simulink model "usato"  (R2016a)
settings: Solver=ode3  StartTime=0.0  StopTime=200  FixedStep=0.1  RelTol=1e-5
values from neighbouring files (symbols this model uses):
  c = 0.1    [Script.m]
  Kd = 0.9    [Script.m]
  Ki = 0.036    [Script.m]
  Kp = 0.37    [Script.m]
  N = 5    [Script.m]
libraries: simulink x2
(part 1 of 2)
settings Model: Creator=The MathWorks, Inc.  LastModifiedBy=User
settings SolverCC: MaxConsecutiveZCs=100000  ZeroCrossAlgorithm=Adaptive
settings DataIOCC: MaxDataPoints=100000  SaveFormat=Array
settings OptimizationCC: ExpressionDepthLimit=2147483647
settings DebuggingCC: UnderspecifiedInitializationDetection=Classic  MergeDetectMultiDrivingBlocksExec=none  FcnCallInpInsideContextMsg=UseLocalSettings  StateNameClashWarn=warning
settings HardwareCC: ProdBitPerPointer=32  ProdLargestAtomicFloat=None  ProdIntDivRoundTo=Undefined  ProdEndianess=Unspecified  ProdWordSize=32  ProdHWDeviceType=32-bit Generic
settings ModelReferenceCC: PropagateSignalLabelsOutOfModel=off
settings GRTTargetCC: CombineOutputUpdateFcns=off  GRTInterface=on
settings ConfigComp: CovModelRefEnable=Off

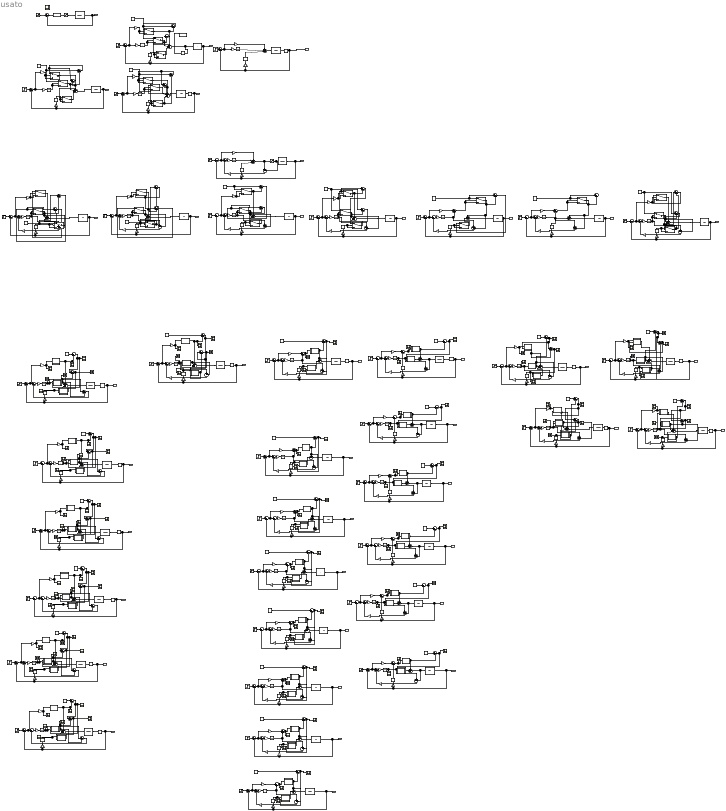
== system usato ==
  note: DESATURAZIONE CLASSICA
  note: TASK P, poi I,poi D
  note: TASK I,poi P,poi D
  note: PI
  note: Anti-Windup PID Control Demonstration
  note: TASK D, poi P,poi I
  note: TASK P, poi D, poi I
  note: TASK I,poi D,poi P
  note: TASK D, poi I,poi P
  note: PD
  note: TASK P, poi I, poi D k=1
  note: PI k=1
  note: PD K=1
  note: TASK I,poi P,poi D
  note: TASK I,poi D,poi P
  note: TASK D, poi P,poi I
  note: TASK D, poi I,poi D
  note: PI k=0.1
  note: PI k=2.8
  note: PI k=2
  note: PI k=3
  note: PI k=0.5
  note: PI k=0.2
  note: PI k=0.75
  note: TASK P, poi I, poi D k=0.1
  note: TASK P, poi I, poi D k=0.2
  note: TASK P, poi I, poi D k=0.5
  note: TASK P, poi I, poi D k=2
  note: TASK P, poi I, poi D k=1,5
  note: PD K=0.1
  note: PD K=0.01
  note: PD K=3
  note: PD K=0.3
  note: PD K=0.03
  C1(t){,1..5} (6 alike) : Constant  Value=c
  Constant{,5..6,10,13..15} (7 alike) : Constant  Value=1.05
  Constant1 : Constant  Value=1.5
  Constant{2,7..9,11..12,16..22} (13 alike) : Constant  Value=c
  Constant3 : Constant  Value=0.1
  Constant4 : Constant  Value=10
  DERIVATIVE{1..37} (37 alike) : Derivative
  Dead Time{,1..14} (15 alike) : TransportDelay  BufferSize=2048
  First Order Process{,2..4,10..12,14..15,19..20} (11 alike) : TransferFcn  Numerator=1  Denominator=[1 1 0]
  First Order Process{1,6,9,16,18} (5 alike) : TransferFcn  Numerator=1  Denominator=[1 0 0]
  First Order Process{5,7,13,17} (4 alike) : TransferFcn  Numerator=1  Denominator=[1 0]
  First Order Process21 : TransferFcn  Numerator=0.1  Denominator=[1 0]
  First Order Process22 : TransferFcn  Numerator=2.8  Denominator=[1 0]
  First Order Process23 : TransferFcn  Numerator=2  Denominator=[1 0]
  First Order Process24 : TransferFcn  Numerator=3  Denominator=[1 0]
  First Order Process25 : TransferFcn  Numerator=0.5  Denominator=[1 0]
  First Order Process26 : TransferFcn  Numerator=0.2  Denominator=[1 0]
  First Order Process27 : TransferFcn  Numerator=0.75  Denominator=[1 0]
  First Order Process28 : TransferFcn  Numerator=0.1  Denominator=[1 1 0]
  First Order Process29 : TransferFcn  Numerator=0.2  Denominator=[1 1 0]
  First Order Process30 : TransferFcn  Numerator=0.5  Denominator=[1 1 0]
  First Order Process31 : TransferFcn  Numerator=2  Denominator=[1 1 0]
  First Order Process32 : TransferFcn  Numerator=1.5  Denominator=[1 1 0]
  First Order Process33 : TransferFcn  Numerator=0.1  Denominator=[1 0 0]
  First Order Process34 : TransferFcn  Numerator=0.01  Denominator=[1 0 0]
  First Order Process35 : TransferFcn  Numerator=3  Denominator=[1 0 0]
  First Order Process36 : TransferFcn  Numerator=100  Denominator=[1 0 0]
  First Order Process37 : TransferFcn  Numerator=0.03  Denominator=[1 0 0]
  First Order Process8 : TransferFcn  Numerator=1  Denominator=[1 1]
  INTEGRATOR{1..25} (25 alike) : Integrator
  Integrator{,1..5} (6 alike) : Integrator
  Kd{1,8,13,17} (4 alike) : Gain  Gain=0
  Kd{4..5,10..12,14..15,19..31} (20 alike) : Gain  Gain=Kd
  Kd{6..7,9,16,18} (5 alike) : Gain  Gain=10
  Kd2 : Gain  Gain=0.9
  Kd3 : Gain  Gain=0.9
  Ki{1,6..9,13,16..18} (9 alike) : Gain  Gain=10
  Ki{4..5,10..12,14..15,19..31} (20 alike) : Gain  Gain=Ki
  Ki2 : Gain  Gain=0.036
  Ki3 : Gain  Gain=0.036
  Kp{1,6..9,13,16..18} (9 alike) : Gain  Gain=10
  Kp{4..5,10..12,14..15,19..31} (20 alike) : Gain  Gain=Kp
  Kp2 : Gain  Gain=0.37
  Kp3 : Gain  Gain=0.37
  MATLAB Function : MATLAB Function  TreatAsAtomicUnit=on
  MATLAB Function1 : MATLAB Function  TreatAsAtomicUnit=on
  MATLAB Function10 : MATLAB Function  TreatAsAtomicUnit=on
  MATLAB Function11 : MATLAB Function  TreatAsAtomicUnit=on
  MATLAB Function12 : MATLAB Function  TreatAsAtomicUnit=on
  MATLAB Function13 : MATLAB Function  TreatAsAtomicUnit=on
  MATLAB Function14 : MATLAB Function  TreatAsAtomicUnit=on
  MATLAB Function15 : MATLAB Function  TreatAsAtomicUnit=on
  MATLAB Function16 : MATLAB Function  TreatAsAtomicUnit=on
  MATLAB Function17 : MATLAB Function  TreatAsAtomicUnit=on
  MATLAB Function18 : MATLAB Function  TreatAsAtomicUnit=on
  MATLAB Function19 : MATLAB Function  TreatAsAtomicUnit=on
  MATLAB Function2 : MATLAB Function  TreatAsAtomicUnit=on
  MATLAB Function20 : MATLAB Function  TreatAsAtomicUnit=on
  MATLAB Function3 : MATLAB Function  TreatAsAtomicUnit=on
  MATLAB Function4 : MATLAB Function  TreatAsAtomicUnit=on
  MATLAB Function5 : MATLAB Function  TreatAsAtomicUnit=on
  MATLAB Function6 : MATLAB Function  TreatAsAtomicUnit=on
  MATLAB Function7 : MATLAB Function  TreatAsAtomicUnit=on
  MATLAB Function8 : MATLAB Function  TreatAsAtomicUnit=on
  MATLAB Function9 : MATLAB Function  TreatAsAtomicUnit=on
  Memory : Memory
  MinMax Running Resettable : simulink/Math Operations/MinMax Running Resettable  Function=max  vinit=0.0
  PID Controller : simulink/Continuous/PID Controller  Controller=PID  TimeDomain=Continuous-time  SampleTime=-1  IntegratorMethod=Forward Euler  FilterMethod=Forward Euler  Form=Parallel  UseFilter=on  ControllerParametersSource=internal  P=Kp  I=Ki  D=Kd  N=N  InitialConditionSource=internal  InitialConditionForIntegrator=0  InitialConditionForFilter=0  ExternalReset=none  LimitOutput=off  UpperSaturationLimit=10  LowerSaturationLimit=-10  LinearizeAsGain=off  AntiWindupMode=none  Kb=1  TrackingMode=off  Kt=1  PParamMin=[]  PParamMax=[]  IParamMin=[]  IParamMax=[]  DParamMin=[]  DParamMax=[]  NParamMin=[]  NParamMax=[]  KbParamMin=[]  KbParamMax=[]  KtParamMin=[]  KtParamMax=[]  POutMin=[]  POutMax=[]  IOutMin=[]  IOutMax=[]  DOutMin=[]  DOutMax=[]  NOutMin=[]  NOutMax=[]  KbOutMin=[]  KbOutMax=[]  KtOutMin=[]  KtOutMax=[]  IntegratorOutMin=[]  IntegratorOutMax=[]  FilterOutMin=[]  FilterOutMax=[]  SumOutMin=[]  SumOutMax=[]  SumI1OutMin=[]  SumI1OutMax=[]  SumI2OutMin=[]  SumI2OutMax=[]  SumI3OutMin=[]  SumI3OutMax=[]  SumDOutMin=[]  SumDOutMax=[]  SaturationOutMin=[]  SaturationOutMax=[]  IntegratorContinuousStateAttributes=''  IntegratorStateMustResolveToSignalObject=off  IntegratorRTWStateStorageClass=Auto  FilterContinuousStateAttributes=''  FilterStateMustResolveToSignalObject=off  FilterRTWStateStorageClass=Auto  DifferentiatorICPrevScaledInput=0  DifferentiatorOutMin=[]  DifferentiatorOutMax=[]
  Saturation : Saturate  UpperLimit=c  LowerLimit=-c
  Saturation1 : Saturate  UpperLimit=c  LowerLimit=-c
  Scope{,1..69} (70 alike) : Scope
  Step{,1..31} (32 alike) : Step  SampleTime=0
  Sum{,1..4,6..10,13..15,17,19..21,23..27,29..31,33..37,39,41,43..45,47..51,53..57,59..61,63..67,69..73,75..79,81..85,87..91,93..99,101..105,107..108,110,112..114,116,118..120,122,124..126,128,130..132,134,136..138,140,142..144,146,148..153,155..159,161..165,167..171,173..177,179..183,185..189,191..195,197..201,203..207,209..210} (165 alike) : Sum  Inputs=|+-
  Sum{5,12,16,18,22,28,32,52,58,62,68,74,80,86,100,106,154,160,166,172,178} (21 alike) : Sum  Inputs=++-|
  Sum{11,38,109,115,121,127,133,139,145} (9 alike) : Sum  Inputs=+-|
  Sum{40,42,111,117,123,129,135,141,147} (9 alike) : Sum  Inputs=|++
  Sum{46,92,184,190,196,202,208} (7 alike) : Sum  Inputs=++|
  Switch{,1..2,9..11,15..17,19..20,28..30,36..41,43} (21 alike) : Switch  Threshold=1.05
  Switch12 : Switch  Threshold=10
  Switch13 : Switch  Threshold=10
  Switch14 : Switch  Threshold=10
  Switch3 : Switch  Threshold=1.5
  Switch4 : Switch  Threshold=1.5
  Switch5 : Switch  Threshold=1.5
  c1(t){,1..5} (6 alike) : Constant  Value=c
  integratore{,1..5} (6 alike) : Integrator
  ka{,1..26} (27 alike) : Gain
  kd{,1..5} (6 alike) : Gain  Gain=Kd
  ki{,1..5} (6 alike) : Gain  Gain=Ki
  kp{,1..5} (6 alike) : Gain  Gain=Kp
  scope{1..42} (42 alike) : Scope
  sigma1 dpi : MATLAB Function  TreatAsAtomicUnit=on
  sigma1 dpi1 : MATLAB Function  TreatAsAtomicUnit=on
  sigma1 idp : MATLAB Function  TreatAsAtomicUnit=on
  sigma1 ipd : MATLAB Function  TreatAsAtomicUnit=on
  sigma1 pd : MATLAB Function  TreatAsAtomicUnit=on
  sigma1 pd1 : MATLAB Function  TreatAsAtomicUnit=on
  sigma1 pd2 : MATLAB Function  TreatAsAtomicUnit=on
  sigma1 pd3 : MATLAB Function  TreatAsAtomicUnit=on
  sigma1 pd4 : MATLAB Function  TreatAsAtomicUnit=on
  sigma1 pd5 : MATLAB Function  TreatAsAtomicUnit=on
  sigma1 pi : MATLAB Function  TreatAsAtomicUnit=on
  sigma1 pi1 : MATLAB Function  TreatAsAtomicUnit=on
  sigma1 pi2 : MATLAB Function  TreatAsAtomicUnit=on
  sigma1 pi3 : MATLAB Function  TreatAsAtomicUnit=on
  sigma1 pi4 : MATLAB Function  TreatAsAtomicUnit=on
  sigma1 pi5 : MATLAB Function  TreatAsAtomicUnit=on
  sigma1 pi6 : MATLAB Function  TreatAsAtomicUnit=on
  sigma1 pi7 : MATLAB Function  TreatAsAtomicUnit=on
  sigma2  idp : MATLAB Function  TreatAsAtomicUnit=on
  sigma2 dpi : MATLAB Function  TreatAsAtomicUnit=on
  sigma2 idp : MATLAB Function  TreatAsAtomicUnit=on
  sigma2 ipd : MATLAB Function  TreatAsAtomicUnit=on
  sigma2 pd : MATLAB Function  TreatAsAtomicUnit=on
  sigma2 pd1 : MATLAB Function  TreatAsAtomicUnit=on
  sigma2 pd2 : MATLAB Function  TreatAsAtomicUnit=on
  sigma2 pd3 : MATLAB Function  TreatAsAtomicUnit=on
  sigma2 pd4 : MATLAB Function  TreatAsAtomicUnit=on
  sigma2 pd5 : MATLAB Function  TreatAsAtomicUnit=on
  sigma2 pi : MATLAB Function  TreatAsAtomicUnit=on
  sigma2 pi1 : MATLAB Function  TreatAsAtomicUnit=on
  sigma2 pi2 : MATLAB Function  TreatAsAtomicUnit=on
  sigma2 pi3 : MATLAB Function  TreatAsAtomicUnit=on
  sigma2 pi4 : MATLAB Function  TreatAsAtomicUnit=on
  sigma2 pi5 : MATLAB Function  TreatAsAtomicUnit=on
  sigma2 pi6 : MATLAB Function  TreatAsAtomicUnit=on
  sigma2 pi7 : MATLAB Function  TreatAsAtomicUnit=on
  sigma3  idp : MATLAB Function  TreatAsAtomicUnit=on
  sigma3  idp1 : MATLAB Function  TreatAsAtomicUnit=on
  sigma3 dpi : MATLAB Function  TreatAsAtomicUnit=on
  sigma3 ipd : MATLAB Function  TreatAsAtomicUnit=on
  step{,1..5} (6 alike) : Step  SampleTime=0
  yout : Outport
  yout5 : Outport  Port=2
  yout2 : Outport  Port=3
  yout6 : Outport  Port=4
  yout1 : Outport  Port=5
  yout4 : Outport  Port=6
  yout7 : Outport  Port=7
  yout8 : Outport  Port=8
  yout9 : Outport  Port=9
  yout13 : Outport  Port=10
  yout14 : Outport  Port=11
  yout16 : Outport  Port=12
  yout17 : Outport  Port=13
  yout18 : Outport  Port=14
  yout15 : Outport  Port=15
  yout3 : Outport  Port=16
  yout10 : Outport  Port=17
  yout11 : Outport  Port=18
  yout20 : Outport  Port=19
  yout12 : Outport  Port=20
  yout19 : Outport  Port=21
  yout21 : Outport  Port=22
  yout22 : Outport  Port=23
  yout23 : Outport  Port=24
  yout24 : Outport  Port=25
  yout25 : Outport  Port=26
  yout26 : Outport  Port=27
  yout27 : Outport  Port=28
  yout28 : Outport  Port=29
  yout29 : Outport  Port=30
  yout30 : Outport  Port=31
  yout31 : Outport  Port=32
  yout32 : Outport  Port=33
  yout33 : Outport  Port=34
  yout34 : Outport  Port=35
  yout35 : Outport  Port=36
  yout36 : Outport  Port=37
  yout37 : Outport  Port=38
  wires:
  Step/1 -> Sum/1  "r(t)"
  Sum/1 -> PID Controller/1  "e(t)"
  First Order Process/1 -> yout/1, Sum/2  "y(t) con saturazione"
  Step5/1 -> Sum10/1  "r(t)"
  Sum10/1 -> Ki1/1, Kp1/1  "e(t)"
  First Order Process5/1 -> yout5/1, Kd1/1, Sum10/2  "yintegrat(t)"
  Ki1/1 -> INTEGRATOR1/1
  Kd1/1 -> DERIVATIVE1/1
  Kp1/1 -> Switch/3, Switch/2
  Switch/1 -> Sum1/2, Sum12/1
  Switch2/1 -> Sum12/3
  DERIVATIVE1/1 -> Switch2/2, Switch2/3
  INTEGRATOR1/1 -> Switch1/3, Switch1/2  "u(t)"
  Switch1/1 -> Sum2/2, Sum12/2
  Sum2/1 -> Switch2/1
  Step2/1 -> Sum14/1  "r(t)"
  Sum14/1 -> Ki3/1, Kp3/1  "e(t)"
  Ki3/1 -> INTEGRATOR3/1
  Kd3/1 -> DERIVATIVE3/1
  INTEGRATOR3/1 -> Sum16/2  "u(t)"
  Kp3/1 -> Sum16/1
  DERIVATIVE3/1 -> Sum16/3
  PID Controller/1 -> Saturation/1  "u(t)"
  Saturation/1 -> First Order Process/1
  Sum12/1 -> Memory/1, First Order Process5/1  "u(t)"
  Step6/1 -> Sum26/1  "r(t)"
  Sum26/1 -> Ki6/1, Kp6/1  "e(t)"
  First Order Process6/1 -> yout6/1, Kd6/1, Sum26/2  "yint(t)"
  Ki6/1 -> INTEGRATOR6/1
  Kd6/1 -> DERIVATIVE6/1
  Constant4/1 -> Switch13/1, Sum25/1
  Kp6/1 -> Switch12/3, Switch12/2
  Switch14/1 -> Sum28/3
  DERIVATIVE6/1 -> Switch14/2, Switch14/3
  INTEGRATOR6/1 -> Switch13/3, Switch13/2  "u(t)"
  Sum30/1 -> Switch14/1
  Sum25/1 -> Sum30/1, Switch12/1
  Switch13/1 -> Sum25/2, Sum28/2
  Switch12/1 -> Sum30/2, Sum28/1
  Sum28/1 -> First Order Process6/1  "u(t)"
  Step1/1 -> Sum4/1  "r(t)"
  Sum4/1 -> Ki2/1, Kp2/1  "e(t)"
  First Order Process1/1 -> Dead Time1/1  "yder(t)"
  Ki2/1 -> INTEGRATOR2/1
  Kd2/1 -> DERIVATIVE2/1
  Kp2/1 -> Switch3/3, Switch3/2
  Switch5/1 -> Sum3/2, Sum5/3
  DERIVATIVE2/1 -> Switch5/2, Switch5/3
  INTEGRATOR2/1 -> Switch4/3, Switch4/2  "u(t)"
  Switch4/1 -> Sum5/2
  Switch3/1 -> Sum6/2, Sum5/1
  Sum5/1 -> First Order Process1/1  "u(t)"
  Constant1/1 -> Sum3/1, Switch5/1
  Sum3/1 -> Switch3/1, Sum6/1
  Sum6/1 -> Switch4/1
  Sum16/1 -> First Order Process2/1  "u(t)"
  First Order Process2/1 -> Dead Time/1  "yrit(t)"
  Dead Time/1 -> yout2/1, Kd3/1, Sum14/2
  Dead Time1/1 -> yout1/1, Kd2/1, Sum4/2
  Memory/1 -> MinMax Running Resettable/1
  Sum1/1 -> Switch/1
  Constant/1 -> Sum1/1, Switch1/1
  Step4/1 -> Sum17/1  "r(t)"
  Sum17/1 -> Sum13/1, Kp5/1  "e(t)"
  First Order Process4/1 -> yout4/1, Kd5/1, Sum17/2  "y(t) con schema di desaturazione classico"
  Ki5/1 -> INTEGRATOR5/1
  Kd5/1 -> DERIVATIVE5/1
  Sum18/1 -> Sum15/1, Saturation1/1  "u(t)"
  Sum13/1 -> Ki5/1
  Saturation1/1 -> Sum15/2, First Order Process4/1
  Sum15/1 -> ka/1
  DERIVATIVE5/1 -> Sum18/3
  INTEGRATOR5/1 -> Sum18/2  "u(t)"
  Kp5/1 -> Sum18/1
  ka/1 -> Sum13/2
  Step7/1 -> Sum21/1  "r(t)"
  Sum21/1 -> Sum19/1, Kp7/1  "e(t)"
  First Order Process7/1 -> yout7/1, Kd7/1, Sum21/2  "ydesat_taskP, poi I, poi D(t)"
  Ki7/1 -> INTEGRATOR7/1
  Kd7/1 -> DERIVATIVE7/1
  Sum22/1 -> First Order Process7/1  "u(t)"
  Sum19/1 -> Ki7/1
  Sum20/1 -> ka1/1
  INTEGRATOR7/1 -> Sum20/1, Switch10/3, Switch10/2  "u(t)"
  Kp7/1 -> Switch9/2, Switch9/3
  ka1/1 -> Sum19/2
  Constant3/1 -> Sum23/1, Switch9/1
  Switch9/1 -> Sum23/2, Sum22/1
  Sum23/1 -> Sum24/1, Switch10/1
  Switch10/1 -> Sum24/2, Sum22/2, Sum20/2
  DERIVATIVE7/1 -> Switch11/2, Switch11/3
  Sum24/1 -> Switch11/1
  Switch11/1 -> Sum22/3
  Step8/1 -> Sum31/1  "r(t)"
  Sum31/1 -> Sum27/1, Kp8/1  "e(t)"
  First Order Process8/1 -> yout8/1, Kd8/1, Sum31/2  "ydesat_task_I,poi P,poi D(t)"
  Ki8/1 -> INTEGRATOR8/1
  Kd8/1 -> DERIVATIVE8/1
  Sum32/1 -> First Order Process8/1  "u(t)"
  Sum27/1 -> Ki8/1
  Sum29/1 -> ka2/1
  INTEGRATOR8/1 -> Sum29/1, Switch15/3, Switch15/2  "u(t)"
  Kp8/1 -> Switch17/2, Switch17/3
  ka2/1 -> Sum27/2
  Switch17/1 -> Sum33/2, Sum32/1
  DERIVATIVE8/1 -> Switch16/2, Switch16/3
  Switch16/1 -> Sum32/3
  Constant5/1 -> Sum34/1, Switch15/1
  Sum34/1 -> Sum33/1, Switch17/1
  Sum33/1 -> Switch16/1
  Step9/1 -> Sum37/1  "r(t)"
  Sum37/1 -> Sum35/1, Kp9/1  "e(t)"
  First Order Process9/1 -> yout9/1, Kd9/1, Sum37/2  "y(t)desatPI"
  Ki9/1 -> INTEGRATOR9/1
  Kd9/1 -> DERIVATIVE9/1
  Sum35/1 -> Ki9/1
  Sum36/1 -> ka3/1
  ka3/1 -> Sum35/2
  DERIVATIVE9/1 -> Switch19/2, Switch19/3
  Switch19/1 -> Sum38/2
  INTEGRATOR9/1 -> Sum36/1, Sum40/2  "u(t)"
  Kp9/1 -> Sum40/1
  Sum40/1 -> Switch20/3, Switch20/2
  Constant6/1 -> Sum39/1, Switch20/1
  Switch20/1 -> Sum39/2, Sum36/2, Sum38/1
  Sum39/1 -> Switch19/1
  Switch15/1 -> Sum34/2, Sum29/2, Sum32/2
  Sum38/1 -> First Order Process9/1  "u(t)"
  Step13/1 -> Sum61/1  "r(t)"
  Sum61/1 -> Sum59/1, Kp13/1  "e(t)"
  First Order Process13/1 -> yout13/1, Kd13/1, Sum61/2  "ydesat_taskD,poi P,poi I(t)"
  Ki13/1 -> INTEGRATOR13/1
  Kd13/1 -> DERIVATIVE13/1
  Sum62/1 -> First Order Process13/1  "u(t)"
  Sum59/1 -> Ki13/1
  Sum60/1 -> ka7/1
  INTEGRATOR13/1 -> Sum60/1, Switch28/3, Switch28/2  "u(t)"
  Kp13/1 -> Switch30/2, Switch30/3
  ka7/1 -> Sum59/2
  Switch30/1 -> Sum64/2, Sum62/1
  Switch28/1 -> Sum62/2, Sum60/2
  DERIVATIVE13/1 -> Switch29/2, Switch29/3
  Switch29/1 -> Sum63/2, Sum62/3
  Constant10/1 -> Sum63/1, Switch29/1
  Sum63/1 -> Switch30/1, Sum64/1
  Sum64/1 -> Switch28/1
  Step14/1 -> Sum67/1  "r(t)"
  Sum67/1 -> Sum65/1, Kp14/1  "e(t)"
  First Order Process14/1 -> Dead Time5/1  "y(t) con tasks nell'ordine:P,D,I"
  Ki14/1 -> INTEGRATOR14/1
  Kd14/1 -> DERIVATIVE14/1
  Sum68/1 -> First Order Process14/1  "u(t)"
  Sum65/1 -> Ki14/1
  Sum66/1 -> ka8/1
  Kp14/1 -> Scope4/1, MATLAB Function/1(qp)
  ka8/1 -> Sum65/2
  Constant11/1 -> Sum69/1
  Sum69/1 -> Scope2/1, MATLAB Function1/2(X), Sum70/1  "c"
  Sum70/1 -> MATLAB Function2/2(Y), Scope3/1
  Step16/1 -> Sum79/1  "r(t)"
  Sum79/1 -> Sum77/1, Kp16/1  "e(t)"
  First Order Process16/1 -> yout16/1, Kd16/1, Sum79/2  "ydesat_task_I,poi D,poi P(t)"
  Ki16/1 -> INTEGRATOR16/1
  Kd16/1 -> DERIVATIVE16/1
  Sum80/1 -> First Order Process16/1  "u(t)"
  Sum77/1 -> Ki16/1
  Sum78/1 -> ka10/1
  INTEGRATOR16/1 -> Sum78/1, Switch36/3, Switch36/2  "u(t)"
  Kp16/1 -> Switch38/2, Switch38/3
  ka10/1 -> Sum77/2
  Switch38/1 -> Sum80/1
  DERIVATIVE16/1 -> Switch37/2, Switch37/3
  Switch37/1 -> Sum81/2, Sum80/3
  Constant13/1 -> Sum82/1, Switch36/1
  Switch36/1 -> Sum82/2, Sum78/2, Sum80/2
  Sum82/1 -> Switch37/1, Sum81/1
  Sum81/1 -> Switch38/1
  Step17/1 -> Sum85/1  "r(t)"
  Sum85/1 -> Sum83/1, Kp17/1  "e(t)"
  First Order Process17/1 -> yout17/1, Kd17/1, Sum85/2  "ydesat_taskD,poi I,poi P(t)"
  Ki17/1 -> INTEGRATOR17/1
  Kd17/1 -> DERIVATIVE17/1
  Sum86/1 -> First Order Process17/1  "u(t)"
  Sum83/1 -> Ki17/1
  Sum84/1 -> ka11/1
  INTEGRATOR17/1 -> Sum84/1, Switch39/3, Switch39/2  "u(t)"
  Kp17/1 -> Switch41/2, Switch41/3
  ka11/1 -> Sum83/2
  Switch41/1 -> Sum86/1
  Switch39/1 -> Sum88/2, Sum86/2, Sum84/2
  DERIVATIVE17/1 -> Switch40/2, Switch40/3
  Switch40/1 -> Sum86/3, Sum87/2
  Constant14/1 -> Sum87/1, Switch40/1
  Sum87/1 -> Sum88/1, Switch39/1
  Sum88/1 -> Switch41/1
  Step18/1 -> Sum91/1  "r(t)"
  Sum91/1 -> Sum89/1, Kp18/1  "e(t)"
  First Order Process18/1 -> yout18/1, Kd18/1, Sum91/2  "y(t)desatPD SENZA I"
  Ki18/1 -> INTEGRATOR18/1
  Kd18/1 -> DERIVATIVE18/1
  Sum89/1 -> Ki18/1
  Sum90/1 -> ka12/1
  ka12/1 -> Sum89/2
  INTEGRATOR18/1 -> Sum92/2, Sum90/1  "u(t)"
  Kp18/1 -> Sum94/1
  Sum94/1 -> Switch43/3, Switch43/2
  Constant15/1 -> Sum93/1, Switch43/1
  Switch43/1 -> Sum93/2, Sum90/2, Sum92/1
  Sum92/1 -> First Order Process18/1  "u(t)"
  DERIVATIVE18/1 -> Sum94/2
  MATLAB Function/1(qpsigma) -> Scope5/1, Sum69/2, Sum68/1
  DERIVATIVE14/1 -> Scope6/1, MATLAB Function1/1(qd)
  MATLAB Function1/1(qdsigma) -> Sum68/3, Sum70/2
  INTEGRATOR14/1 -> Sum66/1, Scope7/1, MATLAB Function2/1(qi)  "u(t)"
  MATLAB Function2/1(qisigma) -> Sum68/2, Sum66/2
  step/1 -> Sum73/1  "r(t)"
  Sum73/1 -> kp/1, Sum71/1  "e(t)"
  First Order Process15/1 -> Dead Time2/1  "y(t) con tasks nell'ordine:P,I,D k=1"
  ki/1 -> integratore/1
  kd/1 -> DERIVATIVE15/1
  Sum74/1 -> First Order Process15/1  "u(t)"
  C1(t)/1 -> Sum75/1
  Sum75/1 -> scope1/1, MATLAB Function5/2(X2), Sum76/1  "C2(t)"
  Sum76/1 -> MATLAB Function4/2(Y2), scope2/1  "C3(t)"
  MATLAB Function3/1(qpsigma) -> scope5/1, Sum75/2, Sum74/1  "Qp ∙σ"
  DERIVATIVE15/1 -> scope3/1, MATLAB Function4/1(qd)  "Qd(t)"
  MATLAB Function4/1(qdsigma) -> Sum74/3  "Qd ∙σ"
  integratore/1 -> Sum72/1, MATLAB Function5/1(qi), scope7/1  "Qi(t)"
  MATLAB Function5/1(qisigma) -> Sum72/2, Sum74/2, scope4/1, Sum76/2  "Qi ∙σ"
  Sum71/1 -> ki/1
  Sum72/1 -> Sum71/2
  kp/1 -> scope6/1, MATLAB Function3/1(qp)  "Qp(t)"
  Step3/1 -> Sum9/1  "r(t)"
  Sum9/1 -> Sum7/1, Kp4/1  "e(t)"
  First Order Process3/1 -> Dead Time3/1  "y(t) con tasks nell'ordine:PI,D K=1"
  Ki4/1 -> INTEGRATOR4/1
  Kd4/1 -> DERIVATIVE4/1
  Sum7/1 -> Ki4/1
  Sum8/1 -> ka4/1
  ka4/1 -> Sum7/2
  INTEGRATOR4/1 -> Sum8/1, Sum42/2  "u(t)"
  Kp4/1 -> Sum42/1
  Constant2/1 -> Sum41/1
  Sum11/1 -> First Order Process3/1  "u(t)"
  Sum42/1 -> Scope14/1, sigma1 pi/1(q_pi)
  sigma1 pi/1(qpisigma) -> Sum41/2, Sum8/2, Sum11/1
  DERIVATIVE4/1 -> Scope16/1, sigma2 pi/1(q_pi_d)
  Sum41/1 -> sigma2 pi/2(Qpi), Scope17/1
  sigma2 pi/1(qpi_dsigma) -> Sum11/2
  Step10/1 -> Sum45/1  "r(t)"
  Sum45/1 -> Sum43/1, Kp10/1  "e(t)"
  First Order Process10/1 -> Dead Time4/1  "y(t) con tasks nell'ordine:PD,I k=1"
  Ki10/1 -> Integrator/1
  Kd10/1 -> DERIVATIVE10/1
  Sum43/1 -> Ki10/1
  Sum44/1 -> ka5/1
  ka5/1 -> Sum43/2
  Integrator/1 -> sigma2 pd/1(q_pd_i), Sum44/1, Scope19/1  "qi(t)"
  Kp10/1 -> Sum48/1  "qp(t)"
  c1(t)/1 -> Sum47/1
  Sum46/1 -> Sum44/2, First Order Process10/1  "u(t)"
  DERIVATIVE10/1 -> Sum48/2  "qd(t)"
  Sum48/1 -> sigma1 pd/1(q_pd), Scope18/1  "qpd(t)"
  sigma1 pd/1(qpdisigma) -> Sum46/1, Sum47/2  "qpd∙σ"
  sigma2 pd/1(qpd_isigma) -> Sum46/2  "qi∙σ"
  Sum47/1 -> sigma2 pd/2(Qpd), Scope20/1  "c2(t)"
  Step11/1 -> Sum51/1  "r(t)"
  Sum51/1 -> Sum49/1, Kp11/1  "e(t)"
  First Order Process11/1 -> Dead Time8/1  "y(t) con tasks nell'ordine:I,P,D"
  Ki11/1 -> INTEGRATOR11/1
  Kd11/1 -> DERIVATIVE11/1
  Sum52/1 -> First Order Process11/1  "u(t)"
  Sum49/1 -> Ki11/1
  Sum50/1 -> ka6/1
  INTEGRATOR11/1 -> sigma1 ipd/1(q_i), Sum50/1, Scope21/1  "u(t)"
  ka6/1 -> Sum49/2
  sigma1 ipd/1(qisigma) -> Sum52/2, Sum53/2, Sum50/2
  Constant8/1 -> Sum53/1
  Kp11/1 -> Scope22/1, sigma2 ipd/1(q_i_p)
  Sum53/1 -> Sum54/1, sigma2 ipd/2(Q_i_p), Scope23/1
  sigma2 ipd/1(q_i_Psigma) -> Sum52/1, Sum54/2
  Sum54/1 -> Scope25/1, sigma3 ipd/2(Q_i_p_d)
  DERIVATIVE11/1 -> Scope24/1, sigma3 ipd/1(q_i_p_d)
  sigma3 ipd/1(q_i_P_dsigma) -> Sum52/3
  Step20/1 -> Sum105/1  "r(t)"
  Sum105/1 -> Sum103/1, Kp20/1  "e(t)"
  First Order Process20/1 -> Dead Time9/1  "y(t) con tasks nell'ordine:I,D,P"
  Ki20/1 -> INTEGRATOR20/1
  Kd20/1 -> DERIVATIVE20/1
  Sum106/1 -> First Order Process20/1  "u(t)"
  Sum103/1 -> Ki20/1
  Sum104/1 -> ka14/1
  INTEGRATOR20/1 -> sigma1 idp/1(q_i3), Sum104/1, Scope36/1  "u(t)"
  ka14/1 -> Sum103/2
  sigma1 idp/1(qi3sigma) -> Sum106/2, Sum107/2, Sum104/2
  Constant17/1 -> Sum107/1
  Kp20/1 -> Scope37/1, sigma3  idp/1(q_i_d_p)
  Sum107/1 -> Sum108/1, sigma2 idp/2(Q_i_d), Scope38/1
  sigma3  idp/1(q_i_d_Psigma) -> Sum106/1
  Sum108/1 -> sigma3  idp/2(Q_i_d_p), Scope40/1
  DERIVATIVE20/1 -> Scope39/1, sigma2 idp/1(q_i_d3)
  sigma2 idp/1(q_i_d_sigma) -> Sum108/2, Sum106/3
  Step12/1 -> Sum57/1  "r(t)"
  Sum57/1 -> Sum55/1, Kp12/1  "e(t)"
  First Order Process12/1 -> Dead Time10/1  "y(t) con tasks nell'ordine:D,P,I"
  Ki12/1 -> INTEGRATOR12/1
  Kd12/1 -> DERIVATIVE12/1
  Sum58/1 -> First Order Process12/1  "u(t)"
  Sum55/1 -> Ki12/1
  Sum56/1 -> ka9/1
  INTEGRATOR12/1 -> Scope34/1, sigma3  idp1/1(q_d_p_i), Sum56/1  "u(t)"
  ka9/1 -> Sum55/2
  Constant9/1 -> Sum95/1
  Sum95/1 -> sigma2 dpi/2(Q_d_p), Sum96/1, Scope27/1
  DERIVATIVE12/1 -> Scope26/1, sigma1 dpi/1(q_d)
  sigma1 dpi/1(qdsigma) -> Sum58/3, Sum95/2
  Kp12/1 -> Scope28/1, sigma2 dpi/1(q_d_p)
  sigma2 dpi/1(q_d_psigma) -> Sum58/1, Sum96/2
  sigma3  idp1/1(q_d_p_isigma) -> Sum56/2, Sum58/2
  Sum96/1 -> Scope29/1, sigma3  idp1/2(Q_d_p_i)
  Step19/1 -> Sum99/1  "r(t)"
  Sum99/1 -> Sum97/1, Kp19/1  "e(t)"
  First Order Process19/1 -> Dead Time11/1  "y(t) con tasks nell'ordine:D,I,P"
  Ki19/1 -> INTEGRATOR19/1
  Kd19/1 -> DERIVATIVE19/1
  Sum100/1 -> First Order Process19/1  "u(t)"
  Sum97/1 -> Ki19/1
  Sum98/1 -> ka13/1
  INTEGRATOR19/1 -> Scope35/1, sigma2  idp/1(q_d_i), Sum98/1  "u(t)"
  ka13/1 -> Sum97/2
  Constant16/1 -> Sum101/1
  DERIVATIVE19/1 -> Scope30/1, sigma1 dpi1/1(q_d1)
  sigma1 dpi1/1(qd1sigma) -> Sum100/3, Sum101/2
  Kp19/1 -> Scope32/1, sigma3 dpi/1(q_d_i_p)
  sigma3 dpi/1(q_d_i_psigma) -> Sum100/1
  sigma2  idp/1(q_d_isigma) -> Sum102/2, Sum98/2, Sum100/2
  Sum102/1 -> sigma3 dpi/2(Q_d_i_p), Scope33/1
  Sum101/1 -> sigma2  idp/2(Q_d_i), Sum102/1, Scope31/1
  Dead Time5/1 -> yout14/1, Kd14/1, Sum67/2
  Dead Time8/1 -> yout11/1, Kd11/1, Sum51/2
  Dead Time9/1 -> yout20/1, Kd20/1, Sum105/2
  Dead Time10/1 -> yout12/1, Kd12/1, Sum57/2
  Dead Time11/1 -> yout19/1, Kd19/1, Sum99/2
  Step15/1 -> Sum114/1  "r(t)"
  Sum114/1 -> Sum112/1, Kp15/1  "e(t)"
  First Order Process21/1 -> yout21/1, Kd15/1, Sum114/2  "y(t) con tasks nell'ordine:PI,D K=0.1"
  Ki15/1 -> INTEGRATOR10/1
  Kd15/1 -> DERIVATIVE21/1
  Sum112/1 -> Ki15/1
  Sum113/1 -> ka15/1
  ka15/1 -> Sum112/2
  INTEGRATOR10/1 -> Sum113/1, Sum111/2  "u(t)"
  Kp15/1 -> Sum111/1
  Constant7/1 -> Sum110/1
  Sum109/1 -> First Order Process21/1  "u(t)"
  Sum111/1 -> Scope8/1, sigma1 pi1/1(qpi_k01)
  sigma1 pi1/1(qpi_k01sigma) -> Sum110/2, Sum113/2, Sum109/1
  DERIVATIVE21/1 -> Scope9/1, sigma2 pi1/1(qpi_d_k01)
  Sum110/1 -> sigma2 pi1/2(C2), Scope10/1
  sigma2 pi1/1(qpi_d_k01sigma) -> Sum109/2
  Step21/1 -> Sum120/1  "r(t)"
  Sum120/1 -> Sum118/1, Kp21/1  "e(t)"
  First Order Process22/1 -> yout22/1, Kd21/1, Sum120/2  "y(t) con tasks nell'ordine:PI,D K=2.8"
  Ki21/1 -> INTEGRATOR15/1
  Kd21/1 -> DERIVATIVE22/1
  Sum118/1 -> Ki21/1
  Sum119/1 -> ka16/1
  ka16/1 -> Sum118/2
  INTEGRATOR15/1 -> Sum119/1, Sum117/2  "u(t)"
  Kp21/1 -> Sum117/1
  Constant12/1 -> Sum116/1
  Sum115/1 -> First Order Process22/1  "u(t)"
  Sum117/1 -> Scope12/1, sigma1 pi2/1(qpi_k10)
  sigma1 pi2/1(qpi_k10sigma) -> Sum116/2, Sum119/2, Sum115/1
  DERIVATIVE22/1 -> Scope13/1, sigma2 pi2/1(qpi_d_k01)
  Sum116/1 -> sigma2 pi2/2(C2k10), Scope11/1
  sigma2 pi2/1(qpi_d_k01sigma) -> Sum115/2
  Step22/1 -> Sum126/1  "r(t)"
  Sum126/1 -> Sum124/1, Kp22/1  "e(t)"
  First Order Process23/1 -> yout23/1, Kd22/1, Sum126/2  "y(t) con tasks nell'ordine:PI,D K=2"
  Ki22/1 -> INTEGRATOR21/1
  Kd22/1 -> DERIVATIVE23/1
  Sum124/1 -> Ki22/1
  Sum125/1 -> ka17/1
  ka17/1 -> Sum124/2
  INTEGRATOR21/1 -> Sum125/1, Sum123/2  "u(t)"
  Kp22/1 -> Sum123/1
  Constant18/1 -> Sum122/1
  Sum121/1 -> First Order Process23/1  "u(t)"
  Sum123/1 -> Scope41/1, sigma1 pi3/1(qpi_k2)
  sigma1 pi3/1(qpi_k2sigma) -> Sum122/2, Sum125/2, Sum121/1
  DERIVATIVE23/1 -> Scope42/1, sigma2 pi3/1(qpi_d_k2)
  Sum122/1 -> sigma2 pi3/2(C2k2), Scope15/1
  sigma2 pi3/1(qpi_d_k2sigma) -> Sum121/2
  Step23/1 -> Sum132/1  "r(t)"
  Sum132/1 -> Sum130/1, Kp23/1  "e(t)"
  First Order Process24/1 -> yout24/1, Kd23/1, Sum132/2  "y(t) con tasks nell'ordine:PI,D K=3"
  Ki23/1 -> INTEGRATOR22/1
  Kd23/1 -> DERIVATIVE24/1
  Sum130/1 -> Ki23/1
  Sum131/1 -> ka18/1
  ka18/1 -> Sum130/2
  INTEGRATOR22/1 -> Sum131/1, Sum129/2  "u(t)"
  Kp23/1 -> Sum129/1
  Constant19/1 -> Sum128/1
  Sum127/1 -> First Order Process24/1  "u(t)"
  Sum129/1 -> Scope44/1, sigma1 pi4/1(qpi_k3)
  sigma1 pi4/1(qpi_k3sigma) -> Sum128/2, Sum131/2, Sum127/1
  DERIVATIVE24/1 -> Scope45/1, sigma2 pi4/1(qpi_d_k3)
  Sum128/1 -> sigma2 pi4/2(C2k3), Scope43/1
  sigma2 pi4/1(qpi_d_k3sigma) -> Sum127/2
  Step24/1 -> Sum138/1  "r(t)"
  Sum138/1 -> Sum136/1, Kp24/1  "e(t)"
  First Order Process25/1 -> yout25/1, Kd24/1, Sum138/2  "y(t) con tasks nell'ordine:PI,D K=0.5"
  Ki24/1 -> INTEGRATOR23/1
  Kd24/1 -> DERIVATIVE25/1
  Sum136/1 -> Ki24/1
  Sum137/1 -> ka19/1
  ka19/1 -> Sum136/2
  INTEGRATOR23/1 -> Sum137/1, Sum135/2  "u(t)"
  Kp24/1 -> Sum135/1
  Constant20/1 -> Sum134/1
  Sum133/1 -> First Order Process25/1  "u(t)"
  Sum135/1 -> Scope47/1, sigma1 pi5/1(qpi_k05)
  sigma1 pi5/1(qpi_k05sigma) -> Sum134/2, Sum137/2, Sum133/1
  DERIVATIVE25/1 -> Scope48/1, sigma2 pi5/1(qpi_d_k05)
  Sum134/1 -> sigma2 pi5/2(C2k05), Scope46/1
  sigma2 pi5/1(qpi_d_k05sigma) -> Sum133/2
  Step25/1 -> Sum144/1  "r(t)"
  Sum144/1 -> Sum142/1, Kp25/1  "e(t)"
  First Order Process26/1 -> yout26/1, Kd25/1, Sum144/2  "y(t) con tasks nell'ordine:PI,D K=0.2"
  Ki25/1 -> INTEGRATOR24/1
  Kd25/1 -> DERIVATIVE26/1
  Sum142/1 -> Ki25/1
  Sum143/1 -> ka20/1
  ka20/1 -> Sum142/2
  INTEGRATOR24/1 -> Sum143/1, Sum141/2  "u(t)"
  Kp25/1 -> Sum141/1
  Constant21/1 -> Sum140/1
  Sum139/1 -> First Order Process26/1  "u(t)"
  Sum141/1 -> Scope50/1, sigma1 pi6/1(qpi_k02)
  sigma1 pi6/1(qpi_k02sigma) -> Sum140/2, Sum143/2, Sum139/1
  DERIVATIVE26/1 -> Scope51/1, sigma2 pi6/1(qpi_d_k02)
  Sum140/1 -> sigma2 pi6/2(C2k02), Scope49/1
  sigma2 pi6/1(qpi_d_k02sigma) -> Sum139/2
  Step26/1 -> Sum150/1  "r(t)"
  Sum150/1 -> Sum148/1, Kp26/1  "e(t)"
  First Order Process27/1 -> yout27/1, Kd26/1, Sum150/2  "y(t) con tasks nell'ordine:PI,D K=0.2"
  Ki26/1 -> INTEGRATOR25/1
  Kd26/1 -> DERIVATIVE27/1
  Sum148/1 -> Ki26/1
  Sum149/1 -> ka21/1
  ka21/1 -> Sum148/2
  INTEGRATOR25/1 -> Sum149/1, Sum147/2  "u(t)"
  Kp26/1 -> Sum147/1
  Constant22/1 -> Sum146/1
  Sum145/1 -> First Order Process27/1  "u(t)"
  Sum147/1 -> Scope53/1, sigma1 pi7/1(qpi_k075)
  sigma1 pi7/1(qpi_k075sigma) -> Sum146/2, Sum149/2, Sum145/1
  DERIVATIVE27/1 -> Scope54/1, sigma2 pi7/1(qpi_d_k075)
  Sum146/1 -> sigma2 pi7/2(C2k075), Scope52/1
  sigma2 pi7/1(qpi_d_k075sigma) -> Sum145/2
  step1/1 -> Sum153/1  "r(t)"
  Sum153/1 -> kp1/1, Sum151/1  "e(t)"
  First Order Process28/1 -> Dead Time6/1  "y(t) con tasks nell'ordine:P,I,D k=0.1"
  ki1/1 -> integratore1/1
  kd1/1 -> DERIVATIVE28/1
  Sum154/1 -> First Order Process28/1  "u(t)"
  C1(t)1/1 -> Sum155/1
  Sum155/1 -> scope8/1, MATLAB Function8/2(c2pk01), Sum156/1  "C2(t)"
  Sum156/1 -> MATLAB Function7/2(c3pk01), scope9/1  "C3(t)"
  MATLAB Function6/1(qpk01sigma) -> scope12/1, Sum155/2, Sum154/1  "Qp ∙σ"
  DERIVATIVE28/1 -> scope10/1, MATLAB Function7/1(qdk01)  "Qd(t)"
  MATLAB Function7/1(qdk01sigma) -> Sum154/3  "Qd ∙σ"
  integratore1/1 -> Sum152/1, MATLAB Function8/1(qik01), scope14/1  "Qi(t)"
  MATLAB Function8/1(qik01sigma) -> Sum152/2, Sum154/2, scope11/1, Sum156/2  "Qi ∙σ"
  Sum151/1 -> ki1/1
  Sum152/1 -> Sum151/2
  kp1/1 -> scope13/1, MATLAB Function6/1(qpk01)  "Qp(t)"
  step2/1 -> Sum159/1  "r(t)"
  Sum159/1 -> kp2/1, Sum157/1  "e(t)"
  First Order Process29/1 -> Dead Time7/1  "y(t) con tasks nell'ordine:P,I,D k=0.2"
  ki2/1 -> integratore2/1
  kd2/1 -> DERIVATIVE29/1
  Sum160/1 -> First Order Process29/1  "u(t)"
  C1(t)2/1 -> Sum161/1
  Sum161/1 -> scope20/1, MATLAB Function11/2(C2pk02), Sum162/1  "C2(t)"
  Sum162/1 -> MATLAB Function10/2(C3pk02), scope21/1  "C3(t)"
  MATLAB Function9/1(qpk02sigma) -> scope17/1, Sum161/2, Sum160/1  "Qp ∙σ"
  DERIVATIVE29/1 -> scope15/1, MATLAB Function10/1(qdk02)  "Qd(t)"
  MATLAB Function10/1(qdk02sigma) -> Sum160/3  "Qd ∙σ"
  integratore2/1 -> Sum158/1, MATLAB Function11/1(qik02), scope19/1  "Qi(t)"
  MATLAB Function11/1(qik02sigma) -> Sum158/2, Sum160/2, scope16/1, Sum162/2  "Qi ∙σ"
  Sum157/1 -> ki2/1
  Sum158/1 -> Sum157/2
  kp2/1 -> scope18/1, MATLAB Function9/1(qpk02)  "Qp(t)"
  step3/1 -> Sum165/1  "r(t)"
  Sum165/1 -> kp3/1, Sum163/1  "e(t)"
  First Order Process30/1 -> Dead Time12/1  "y(t) con tasks nell'ordine:P,I,D k=0.5"
  ki3/1 -> integratore3/1
  kd3/1 -> DERIVATIVE30/1
  Sum166/1 -> First Order Process30/1  "u(t)"
  C1(t)3/1 -> Sum167/1
  Sum167/1 -> scope27/1, MATLAB Function13/2(C2pk05), Sum168/1  "C2(t)"
  Sum168/1 -> MATLAB Function12/2(C3pk05), scope28/1  "C3(t)"
  MATLAB Function14/1(qpk05sigma) -> scope24/1, Sum167/2, Sum166/1  "Qp ∙σ"
  DERIVATIVE30/1 -> scope22/1, MATLAB Function12/1(qdk05)  "Qd(t)"
  MATLAB Function12/1(qdk05sigma) -> Sum166/3  "Qd ∙σ"
  integratore3/1 -> Sum164/1, MATLAB Function13/1(qik05), scope26/1  "Qi(t)"
  MATLAB Function13/1(qik05sigma) -> Sum164/2, Sum166/2, scope23/1, Sum168/2  "Qi ∙σ"
  Sum163/1 -> ki3/1
  Sum164/1 -> Sum163/2
  kp3/1 -> scope25/1, MATLAB Function14/1(qpk05)  "Qp(t)"
  step4/1 -> Sum171/1  "r(t)"
  Sum171/1 -> kp4/1, Sum169/1  "e(t)"
  First Order Process31/1 -> Dead Time13/1  "y(t) con tasks nell'ordine:P,I,D k=2"
  ki4/1 -> integratore4/1
  kd4/1 -> DERIVATIVE31/1
  Sum172/1 -> First Order Process31/1  "u(t)"
  C1(t)4/1 -> Sum173/1
  Sum173/1 -> scope34/1, MATLAB Function16/2(C2pk2), Sum174/1  "C2(t)"
  Sum174/1 -> MATLAB Function15/2(C3pk2), scope35/1  "C3(t)"
  MATLAB Function17/1(qpk2sigma) -> scope31/1, Sum173/2, Sum172/1  "Qp ∙σ"
  DERIVATIVE31/1 -> scope29/1, MATLAB Function15/1(qdk2)  "Qd(t)"
  MATLAB Function15/1(qdk2sigma) -> Sum172/3  "Qd ∙σ"
  integratore4/1 -> Sum170/1, MATLAB Function16/1(qik2), scope33/1  "Qi(t)"
  MATLAB Function16/1(qik2sigma) -> Sum170/2, Sum172/2, scope30/1, Sum174/2  "Qi ∙σ"
  Sum169/1 -> ki4/1
  Sum170/1 -> Sum169/2
  kp4/1 -> scope32/1, MATLAB Function17/1(qpk2)  "Qp(t)"
  step5/1 -> Sum177/1  "r(t)"
  Sum177/1 -> kp5/1, Sum175/1  "e(t)"
  First Order Process32/1 -> Dead Time14/1  "y(t) con tasks nell'ordine:P,I,D k=1.5"
  ki5/1 -> integratore5/1
  kd5/1 -> DERIVATIVE32/1
  Sum178/1 -> First Order Process32/1  "u(t)"
  C1(t)5/1 -> Sum179/1
  Sum179/1 -> scope41/1, MATLAB Function19/2(C2pk26), Sum180/1  "C2(t)"
  Sum180/1 -> MATLAB Function18/2(C3pk26), scope42/1  "C3(t)"
  MATLAB Function20/1(qpk26sigma) -> scope38/1, Sum179/2, Sum178/1  "Qp ∙σ"
  DERIVATIVE32/1 -> scope36/1, MATLAB Function18/1(qdk26)  "Qd(t)"
  MATLAB Function18/1(qdk26sigma) -> Sum178/3  "Qd ∙σ"
  integratore5/1 -> Sum176/1, MATLAB Function19/1(qik26), scope40/1  "Qi(t)"
  MATLAB Function19/1(qik26sigma) -> Sum176/2, Sum178/2, scope37/1, Sum180/2  "Qi ∙σ"
  Sum175/1 -> ki5/1
  Sum176/1 -> Sum175/2
  kp5/1 -> scope39/1, MATLAB Function20/1(qpk26)  "Qp(t)"
  Step27/1 -> Sum183/1  "r(t)"
  Sum183/1 -> Sum181/1, Kp27/1  "e(t)"
  First Order Process33/1 -> yout33/1, Kd27/1, Sum183/2  "y(t) con tasks nell'ordine:PD,I k=0.1"
  Ki27/1 -> Integrator1/1
  Kd27/1 -> DERIVATIVE33/1
  Sum181/1 -> Ki27/1
  Sum182/1 -> ka22/1
  ka22/1 -> Sum181/2
  Integrator1/1 -> sigma2 pd1/1(qi01), Sum182/1, Scope56/1  "qi(t)"
  Kp27/1 -> Sum186/1  "qp(t)"
  c1(t)1/1 -> Sum185/1
  Sum184/1 -> Sum182/2, First Order Process33/1  "u(t)"
  DERIVATIVE33/1 -> Sum186/2  "qd(t)"
  Sum186/1 -> sigma1 pd1/1(qpd01), Scope55/1  "qpd(t)"
  sigma1 pd1/1(qpd01sigma) -> Sum184/1, Sum185/2  "qpd∙σ"
  sigma2 pd1/1(qi01sigma) -> Sum184/2  "qi∙σ"
  Sum185/1 -> sigma2 pd1/2(C2pd01), Scope57/1  "c2(t)"
  Step28/1 -> Sum189/1  "r(t)"
  Sum189/1 -> Sum187/1, Kp28/1  "e(t)"
  First Order Process34/1 -> yout34/1, Kd28/1, Sum189/2  "y(t) con tasks nell'ordine:PD,I k=0.01"
  Ki28/1 -> Integrator2/1
  Kd28/1 -> DERIVATIVE34/1
  Sum187/1 -> Ki28/1
  Sum188/1 -> ka23/1
  ka23/1 -> Sum187/2
  Integrator2/1 -> sigma2 pd2/1(qi001), Sum188/1, Scope59/1  "qi(t)"
  Kp28/1 -> Sum192/1  "qp(t)"
  c1(t)2/1 -> Sum191/1
  Sum190/1 -> Sum188/2, First Order Process34/1  "u(t)"
  DERIVATIVE34/1 -> Sum192/2  "qd(t)"
  Sum192/1 -> sigma1 pd2/1(qpd001), Scope58/1  "qpd(t)"
  sigma1 pd2/1(qpd001sigma) -> Sum190/1, Sum191/2  "qpd∙σ"
  sigma2 pd2/1(qi001sigma) -> Sum190/2  "qi∙σ"
  Sum191/1 -> sigma2 pd2/2(C2pd001), Scope60/1  "c2(t)"
  Step29/1 -> Sum195/1  "r(t)"
  Sum195/1 -> Sum193/1, Kp29/1  "e(t)"
  First Order Process35/1 -> yout35/1, Kd29/1, Sum195/2  "y(t) con tasks nell'ordine:PD,I k=3"
  Ki29/1 -> Integrator3/1
  Kd29/1 -> DERIVATIVE35/1
  Sum193/1 -> Ki29/1
  Sum194/1 -> ka24/1
  ka24/1 -> Sum193/2
  Integrator3/1 -> sigma2 pd3/1(qi10), Sum194/1, Scope62/1  "qi(t)"
  Kp29/1 -> Sum198/1  "qp(t)"
  c1(t)3/1 -> Sum197/1
  Sum196/1 -> Sum194/2, First Order Process35/1  "u(t)"
  DERIVATIVE35/1 -> Sum198/2  "qd(t)"
  Sum198/1 -> sigma1 pd3/1(qpd10), Scope61/1  "qpd(t)"
  sigma1 pd3/1(qpd10sigma) -> Sum196/1, Sum197/2  "qpd∙σ"
  sigma2 pd3/1(qi10sigma) -> Sum196/2  "qi∙σ"
  Sum197/1 -> sigma2 pd3/2(C2pd10), Scope63/1  "c2(t)"
  Step30/1 -> Sum201/1  "r(t)"
  Sum201/1 -> Sum199/1, Kp30/1  "e(t)"
  First Order Process36/1 -> yout36/1, Kd30/1, Sum201/2  "y(t) con tasks nell'ordine:PD,I k=0.3"
  Ki30/1 -> Integrator4/1
  Kd30/1 -> DERIVATIVE36/1
  Sum199/1 -> Ki30/1
  Sum200/1 -> ka25/1
  ka25/1 -> Sum199/2
  Integrator4/1 -> sigma2 pd4/1(qi0001), Sum200/1, Scope65/1  "qi(t)"
  Kp30/1 -> Sum204/1  "qp(t)"
  c1(t)4/1 -> Sum203/1
  Sum202/1 -> Sum200/2, First Order Process36/1  "u(t)"
  DERIVATIVE36/1 -> Sum204/2  "qd(t)"
  Sum204/1 -> sigma1 pd4/1(qpd0001), Scope64/1  "qpd(t)"
  sigma1 pd4/1(qpd0001sigma) -> Sum202/1, Sum203/2  "qpd∙σ"
  sigma2 pd4/1(qi0001sigma) -> Sum202/2  "qi∙σ"
  Sum203/1 -> sigma2 pd4/2(C2pd0001), Scope66/1  "c2(t)"
  Step31/1 -> Sum207/1  "r(t)"
  Sum207/1 -> Sum205/1, Kp31/1  "e(t)"
  First Order Process37/1 -> yout37/1, Kd31/1, Sum207/2  "y(t) con tasks nell'ordine:PD,I k=0.03"
  Ki31/1 -> Integrator5/1
  Kd31/1 -> DERIVATIVE37/1
  Sum205/1 -> Ki31/1
  Sum206/1 -> ka26/1
  ka26/1 -> Sum205/2
  Integrator5/1 -> sigma2 pd5/1(qi003), Sum206/1, Scope68/1  "qi(t)"
  Kp31/1 -> Sum210/1  "qp(t)"
  c1(t)5/1 -> Sum209/1
  Sum208/1 -> Sum206/2, First Order Process37/1  "u(t)"
  DERIVATIVE37/1 -> Sum210/2  "qd(t)"
  Sum210/1 -> sigma1 pd5/1(qpd003), Scope67/1  "qpd(t)"
  sigma1 pd5/1(qpd003sigma) -> Sum208/1, Sum209/2  "qpd∙σ"
  sigma2 pd5/1(qi003sigma) -> Sum208/2  "qi∙σ"
  Sum209/1 -> sigma2 pd5/2(C2pd003), Scope69/1  "c2(t)"
  Dead Time2/1 -> yout15/1, kd/1, Sum73/2
  Dead Time3/1 -> yout3/1, Kd4/1, Sum9/2
  Dead Time4/1 -> yout10/1, Kd10/1, Sum45/2
  Dead Time6/1 -> yout28/1, kd1/1, Sum153/2
  Dead Time7/1 -> yout29/1, kd2/1, Sum159/2
  Dead Time12/1 -> yout30/1, kd3/1, Sum165/2
  Dead Time13/1 -> yout31/1, kd4/1, Sum171/2
  Dead Time14/1 -> yout32/1, kd5/1, Sum177/2

== matlab function usato/MATLAB Function1 ==
  data: qd input; qdsigma output; X input
function qdsigma=sigma(qd,X)

    if(qd > X)
        qdsigma=X;
    
    else
        if(qd < -X)
            qdsigma = -X;
        else
        if(qd == 0)
                qdsigma=0;
        else
            qdsigma=qd;
        end
        end
    end

== matlab function usato/MATLAB Function ==
  data: qp input; qpsigma output
function qpsigma=sigma(qp)
    if(qp > 1.05)
        qpsigma=1.05;
    
    else
        if(qp < -1.05)
            qpsigma = -1.05;
        else
        if(qp == 0)
                qpsigma=0;
        else
            qpsigma=qp;
        end
        end
    end

== matlab function usato/MATLAB Function2 ==
  data: qi input; qisigma output; Y input
function qisigma=sigma(qi,Y)
    if(qi > Y)
        qisigma=Y;
    
    else
        if(qi < -Y)
            qisigma = -Y;
        else
        if(qi == 0)
                qisigma=0;
        else
            qisigma=qi;
        end
        end
    end

== matlab function usato/MATLAB Function3 ==
  data: qp input; qpsigma output
function qpsigma=sigma(qp)
    if(qp > 1.05)
        qpsigma=1.05;
    
    else
        if(qp < -1.05)
            qpsigma = -1.05;
        else
        if(qp == 0)
                qpsigma=0;
        else
            qpsigma=qp;
        end
        end
    end

== matlab function usato/MATLAB Function4 ==
  data: qd input; qdsigma output; Y2 input
function qdsigma=sigma(qd,Y2)

    if(qd > Y2)
        qdsigma=Y2;
    
    else
        if(qd < -Y2)
            qdsigma = -Y2;
        else
        if(qd == 0)
                qdsigma=0;
        else
            qdsigma=qd;
        end
        end
    end

== matlab function usato/MATLAB Function5 ==
  data: qi input; qisigma output; X2 input
function qisigma=sigma(qi,X2)
    if(qi > X2)
        qisigma=X2;
    
    else
        if(qi < -X2)
            qisigma = -X2;
        else
        if(qi == 0)
                qisigma=0;
        else
            qisigma=qi;
        end
        end
    end

== matlab function usato/sigma1 pi ==
  data: q_pi input; qpisigma output
function qpisigma=sigma(q_pi)
    if(q_pi > 1.05)
        qpisigma=1.05;
    
    else
        if(q_pi < -1.05)
            qpisigma = -1.05;
        else
        if(q_pi == 0)
                qpisigma=0;
        else
            qpisigma=q_pi;
        end
        end
    end

== matlab function usato/sigma2 pi ==
  data: q_pi_d input; qpi_dsigma output; Qpi input
function qpi_dsigma=sigma(q_pi_d,Qpi)
    if(q_pi_d > Qpi)
        qpi_dsigma=Qpi;
    
    else
        if(q_pi_d < -Qpi)
            qpi_dsigma =-Qpi;
        else
        if(q_pi_d == 0)
                qpi_dsigma=0;
        else
            qpi_dsigma=q_pi_d;
        end
        end
    end

== matlab function usato/sigma1 pd ==
  data: q_pd input; qpdisigma output
function qpdisigma=sigma(q_pd)
    if(q_pd > 1.05)
        qpdisigma=1.05;
    
    else
        if(q_pd < -1.05)
            qpdisigma = -1.05;
        else
        if(q_pd == 0)
                qpdisigma=0;
        else
            qpdisigma=q_pd;
        end
        end
    end

== matlab function usato/sigma2 pd ==
  data: q_pd_i input; qpd_isigma output; Qpd input
function qpd_isigma=sigma(q_pd_i,Qpd)
    if(q_pd_i > Qpd)
        qpd_isigma=Qpd;
    
    else
        if(q_pd_i < -Qpd)
            qpd_isigma = -Qpd;
        else
        if(q_pd_i == 0)
                qpd_isigma=0;
        else
            qpd_isigma=q_pd_i;
        end
        end
    end

== matlab function usato/sigma1 ipd ==
  data: q_i input; qisigma output
function qisigma=sigma(q_i)
    if(q_i > 1.05)
        qisigma=1.05;
    
    else
        if(q_i < -1.05)
            qisigma = -1.05;
        else
        if(q_i == 0)
                qisigma=0;
        else
            qisigma=q_i;
        end
        end
    end

== matlab function usato/sigma2 ipd ==
  data: q_i_p input; q_i_Psigma output; Q_i_p input
function q_i_Psigma=sigma(q_i_p,Q_i_p)
    if(q_i_p > Q_i_p)
        q_i_Psigma=Q_i_p;
    
    else
        if(q_i_p < -Q_i_p)
            q_i_Psigma = -Q_i_p;
        else
        if(q_i_p == 0)
                q_i_Psigma=0;
        else
            q_i_Psigma=q_i_p;
        end
        end
    end

== matlab function usato/sigma3 ipd ==
  data: q_i_p_d input; q_i_P_dsigma output; Q_i_p_d input
function q_i_P_dsigma=sigma(q_i_p_d,Q_i_p_d)
    if(q_i_p_d > Q_i_p_d)
        q_i_P_dsigma=Q_i_p_d;
    
    else
        if(q_i_p_d < -Q_i_p_d)
            q_i_P_dsigma = -Q_i_p_d;
        else
        if(q_i_p_d == 0)
                q_i_P_dsigma=0;
        else
            q_i_P_dsigma=q_i_p_d;
        end
        end
    end

== matlab function usato/sigma1 dpi ==
  data: q_d input; qdsigma output
function qdsigma=sigma(q_d)
    if(q_d > 1.05)
        qdsigma=1.05;
    
    else
        if(q_d < -1.05)
            qdsigma = -1.05;
        else
        if(q_d == 0)
                qdsigma=0;
        else
            qdsigma=q_d;
        end
        end
    end

== matlab function usato/sigma2 dpi ==
  data: q_d_p input; q_d_psigma output; Q_d_p input
function q_d_psigma=sigma(q_d_p,Q_d_p)
    if(q_d_p > Q_d_p)
        q_d_psigma=Q_d_p;
    
    else
        if(q_d_p < -Q_d_p)
            q_d_psigma = -Q_d_p;
        else
        if(q_d_p == 0)
                q_d_psigma=0;
        else
            q_d_psigma=q_d_p;
        end
        end
    end

== matlab function usato/sigma3  idp1 ==
  data: q_d_p_i input; q_d_p_isigma output; Q_d_p_i input
function q_d_p_isigma=sigma(q_d_p_i,Q_d_p_i)
    if(q_d_p_i > Q_d_p_i)
        q_d_p_isigma=Q_d_p_i;
    
    else
        if(q_d_p_i < -Q_d_p_i)
            q_d_p_isigma = -Q_d_p_i;
        else
        if(q_d_p_i == 0)
                q_d_p_isigma=0;
        else
            q_d_p_isigma=q_d_p_i;
        end
        end
    end

== matlab function usato/sigma1 dpi1 ==
  data: q_d1 input; qd1sigma output
function qd1sigma=sigma(q_d1)
    if(q_d1 > 1.05)
        qd1sigma=1.05;
    
    else
        if(q_d1 < -1.05)
            qd1sigma = -1.05;
        else
        if(q_d1 == 0)
                qd1sigma=0;
        else
            qd1sigma=q_d1;
        end
        end
    end

== matlab function usato/sigma3 dpi ==
  data: q_d_i_p input; q_d_i_psigma output; Q_d_i_p input
function q_d_i_psigma=sigma(q_d_i_p,Q_d_i_p)
    if(q_d_i_p > Q_d_i_p)
        q_d_i_psigma=Q_d_i_p;
    
    else
        if(q_d_i_p < -Q_d_i_p)
            q_d_i_psigma = -Q_d_i_p;
        else
        if(q_d_i_p == 0)
                q_d_i_psigma=0;
        else
            q_d_i_psigma=q_d_i_p;
        end
        end
    end

== matlab function usato/sigma2  idp ==
  data: q_d_i input; q_d_isigma output; Q_d_i input
function q_d_isigma=sigma(q_d_i,Q_d_i)
    if(q_d_i > Q_d_i)
        q_d_isigma=Q_d_i;
    
    else
        if(q_d_i < -Q_d_i)
            q_d_isigma = -Q_d_i;
        else
        if(q_d_i == 0)
                q_d_isigma=0;
        else
            q_d_isigma=q_d_i;
        end
        end
    end

== matlab function usato/sigma1 idp ==
  data: q_i3 input; qi3sigma output
function qi3sigma=sigma(q_i3)
    if(q_i3 > 1.05)
        qi3sigma=1.05;
    
    else
        if(q_i3 < -1.05)
            qi3sigma = -1.05;
        else
        if(q_i3 == 0)
                qi3sigma=0;
        else
            qi3sigma=q_i3;
        end
        end
    end

== matlab function usato/sigma3  idp ==
  data: q_i_d_p input; q_i_d_Psigma output; Q_i_d_p input
function q_i_d_Psigma=sigma(q_i_d_p,Q_i_d_p)
    if(q_i_d_p > Q_i_d_p)
        q_i_d_Psigma=Q_i_d_p;
    
    else
        if(q_i_d_p < -Q_i_d_p)
            q_i_d_Psigma = -Q_i_d_p;
        else
        if(q_i_d_p == 0)
                q_i_d_Psigma=0;
        else
            q_i_d_Psigma=q_i_d_p;
        end
        end
    end

== matlab function usato/sigma2 idp ==
  data: q_i_d3 input; q_i_d_sigma output; Q_i_d input
function q_i_d_sigma=sigma(q_i_d3,Q_i_d)
    if(q_i_d3 > Q_i_d)
        q_i_d_sigma=Q_i_d;
    
    else
        if(q_i_d3 < -Q_i_d)
            q_i_d_sigma = -Q_i_d;
        else
        if(q_i_d3 == 0)
                q_i_d_sigma=0;
        else
            q_i_d_sigma=q_i_d3;
        end
        end
    end

== matlab function usato/sigma1 pi1 ==
  data: qpi_k01 input; qpi_k01sigma output
function qpi_k01sigma=sigma(qpi_k01)
    if(qpi_k01 > 1.05)
        qpi_k01sigma=1.05;
    
    else
        if(qpi_k01 < -1.05)
            qpi_k01sigma = -1.05;
        else
        if(qpi_k01 == 0)
                qpi_k01sigma=0;
        else
            qpi_k01sigma=qpi_k01;
        end
        end
    end

== matlab function usato/sigma2 pi1 ==
  data: qpi_d_k01 input; qpi_d_k01sigma output; C2 input
function qpi_d_k01sigma=sigma(qpi_d_k01,C2)
    if(qpi_d_k01 > C2)
        qpi_d_k01sigma=C2;
    
    else
        if(qpi_d_k01 < -C2)
            qpi_d_k01sigma =-C2;
        else
        if(qpi_d_k01 == 0)
                qpi_d_k01sigma=0;
        else
            qpi_d_k01sigma=qpi_d_k01;
        end
        end
    end

== matlab function usato/sigma1 pi2 ==
  data: qpi_k10 input; qpi_k10sigma output
function qpi_k10sigma=sigma(qpi_k10)
    if(qpi_k10 > 1.05)
        qpi_k10sigma=1.05;
    
    else
        if(qpi_k10 < -1.05)
            qpi_k10sigma = -1.05;
        else
        if(qpi_k10 == 0)
                qpi_k10sigma=0;
        else
            qpi_k10sigma=qpi_k10;
        end
        end
    end

== matlab function usato/sigma2 pi2 ==
  data: qpi_d_k01 input; qpi_d_k01sigma output; C2k10 input
function qpi_d_k01sigma=sigma(qpi_d_k01,C2k10)
    if(qpi_d_k01 > C2k10)
        qpi_d_k01sigma=C2k10;
    
    else
        if(qpi_d_k01 < -C2k10)
            qpi_d_k01sigma =-C2k10;
        else
        if(qpi_d_k01 == 0)
                qpi_d_k01sigma=0;
        else
            qpi_d_k01sigma=qpi_d_k01;
        end
        end
    end

== matlab function usato/sigma1 pi3 ==
  data: qpi_k2 input; qpi_k2sigma output
function qpi_k2sigma=sigma(qpi_k2)
    if(qpi_k2 > 1.05)
        qpi_k2sigma=1.05;
    
    else
        if(qpi_k2 < -1.05)
            qpi_k2sigma = -1.05;
        else
        if(qpi_k2 == 0)
                qpi_k2sigma=0;
        else
            qpi_k2sigma=qpi_k2;
        end
        end
    end

== matlab function usato/sigma2 pi3 ==
  data: qpi_d_k2 input; qpi_d_k2sigma output; C2k2 input
function qpi_d_k2sigma=sigma(qpi_d_k2,C2k2)
    if(qpi_d_k2 > C2k2)
        qpi_d_k2sigma=C2k2;
    
    else
        if(qpi_d_k2 < -C2k2)
            qpi_d_k2sigma =-C2k2;
        else
        if(qpi_d_k2 == 0)
                qpi_d_k2sigma=0;
        else
            qpi_d_k2sigma=qpi_d_k2;
        end
        end
    end

== matlab function usato/sigma1 pi4 ==
  data: qpi_k3 input; qpi_k3sigma output
function qpi_k3sigma=sigma(qpi_k3)
    if(qpi_k3 > 1.05)
        qpi_k3sigma=1.05;
    
    else
        if(qpi_k3 < -1.05)
            qpi_k3sigma = -1.05;
        else
        if(qpi_k3 == 0)
                qpi_k3sigma=0;
        else
            qpi_k3sigma=qpi_k3;
        end
        end
    end

== matlab function usato/sigma2 pi4 ==
  data: qpi_d_k3 input; qpi_d_k3sigma output; C2k3 input
function qpi_d_k3sigma=sigma(qpi_d_k3,C2k3)
    if(qpi_d_k3 > C2k3)
        qpi_d_k3sigma=C2k3;
    
    else
        if(qpi_d_k3 < -C2k3)
            qpi_d_k3sigma =-C2k3;
        else
        if(qpi_d_k3 == 0)
                qpi_d_k3sigma=0;
        else
            qpi_d_k3sigma=qpi_d_k3;
        end
        end
    end

== matlab function usato/sigma1 pi5 ==
  data: qpi_k05 input; qpi_k05sigma output
function qpi_k05sigma=sigma(qpi_k05)
    if(qpi_k05 > 1.05)
        qpi_k05sigma=1.05;
    
    else
        if(qpi_k05 < -1.05)
            qpi_k05sigma = -1.05;
        else
        if(qpi_k05 == 0)
                qpi_k05sigma=0;
        else
            qpi_k05sigma=qpi_k05;
        end
        end
    end
